simulink model "lab4"  (R2022b)
settings: Solver=VariableStepAuto  StartTime=0.0  StopTime=0.06  RelTol=1e-3
undefined symbols (not defined in the file): plecs
libraries: simulink x1, modelsimlib x1
settings Model: Creator=qawse  LastModifiedBy=qawse

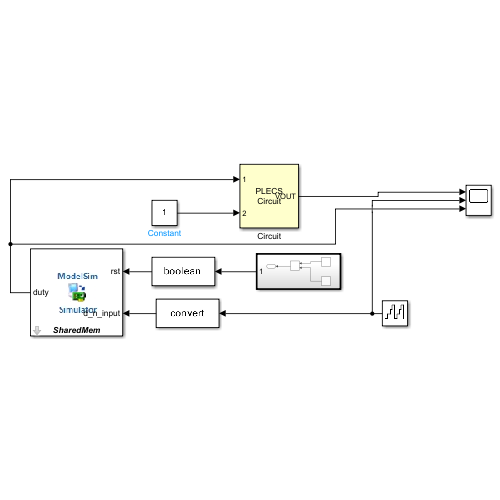
[thumbnail: Simulink's stored preview of the top-level diagram]
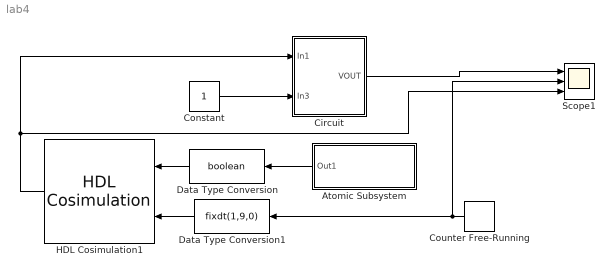
== system lab4 ==
  Atomic Subsystem : Subsystem  TreatAsAtomicUnit=on
  Circuit : Subsystem  LoadFcn=plecs('sl', 200);  InitFcn=plecs('sl', 214);  StartFcn=plecs('sl', 208);  StopFcn=plecs('sl', 209);  mask(PlecsCircuit){PLECSData=<binary blob, 2616 chars, not shown>}
      mask prompts: PLECSData "PLECS Data (Do not delete or modify!)"
      mask init:
      | % PLACE CUSTOM INITIALIZATIONS ABOVE
      | % DO NOT REMOVE
      | plecs('sl', 215);
      | % DO NOT REMOVE
      settings: CopyFcn=plecs('sl', 203);  DeleteFcn=plecs('sl', 205);  UndoDeleteFcn=plecs('sl', 206);  PreSaveFcn=plecs('sl', 211);  PostSaveFcn=plecs('sl', 201);  NameChangeFcn=plecs('sl', 210);  DestroyFcn=plecs('sl', 207);  PreCopyFcn=plecs('sl', 216);  OpenFcn=plecs('sl', 202);  ErrorFcn=plerrorfcn
      mask Help: web(['file:///' fullfile(plecsdoc, 'creatingacircuit.html')])
      mask Display: disp('PLECS\nCircuit')
  Constant : Constant
  Counter Free-Running : simulink/Sources/Counter Free-Running  NumBits=9  tsamp=1e-3
  Data Type Conversion : DataTypeConversion  OutDataTypeStr=boolean  SaturateOnIntegerOverflow=off  RndMeth=Floor
  Data Type Conversion1 : DataTypeConversion  OutDataTypeStr=fixdt(1,9,0)  SaturateOnIntegerOverflow=off  RndMeth=Floor
  HDL Cosimulation1 : modelsimlib/HDL Cosimulation  PortPaths=/counter_dpwm/rst;/counter_dpwm/d_n_input;/counter_dpwm/duty  PortModes=[1 1 2 ]  PortTimes=[-1,-1,4e-9]  PortSigns=[-1 -1 -1 ]  PortFracLengths=[0,0,0]  CommLocal=on  CommSharedMemory=on  CommPortNumber=4449  CommShowInfo=on  ClockPaths=/counter_dpwm/clk  ClockModes=[2 ]  ClockTimes=[4e-9]  TclPreSimCommand="puts \"Running Simulink Cosimulation block.\""  TclPostSimCommand="puts \"done\""  TimingMode=s  TimingScaleFactor=1  idxCellArray={'UNUSED_VAR'}  CosimBypass=Full Simulation  AllowDirectFeedthrough=off  ProductName=EDA Simulator Link MQ  RunAutoTimescale=off  HdlClocks=0  PreRunTime=0  PreRunTimeUnit=ns
  Scope1 : Scope  NumInputPorts=3
  wires:
  Circuit/1(VOUT) -> Scope1/1
  Atomic Subsystem/1(Out1) -> Data Type Conversion/1
  Counter Free-Running/1 -> Data Type Conversion1/1, Scope1/2
  Constant/1 -> Circuit/2(In3)
  Data Type Conversion/1 -> HDL Cosimulation1/1
  Data Type Conversion1/1 -> HDL Cosimulation1/2
  HDL Cosimulation1/1 -> Circuit/1(In1), Scope1/3

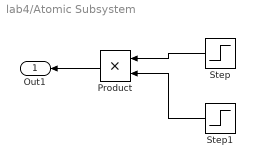
== system lab4/Atomic Subsystem ==
  Product : Product
  Step : Step  Time=1e-6  SampleTime=2e-8
  Step1 : Step  Time=1.6e-6  Before=1  After=0  SampleTime=2e-8
  Out1 : Outport
  wires:
  Product/1 -> Out1/1
  Step/1 -> Product/1
  Step1/1 -> Product/2

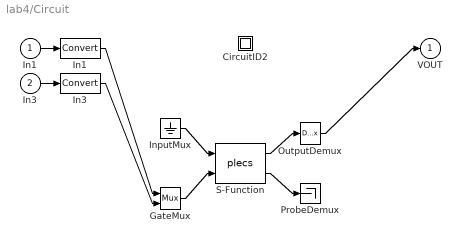
== system lab4/Circuit ==
  In1 : Inport  PortDimensions=1
  In3 : Inport  Port=2  PortDimensions=1
  " CircuitID2 " : Subsystem
  " GateMux " : Mux  Inputs=[ 1 1 ]
  " In1 " : DataTypeConversion
  " In3 " : DataTypeConversion
  " InputMux " : Ground
  " OutputDemux " : Demux  Outputs=[ 1 ]
  " ProbeDemux " : Terminator
  " S-Function " : S-Function  FunctionName=plecs  SFunctionDeploymentMode=off  EnableBusSupport=off
  VOUT : Outport  PortDimensions=1
  wires:
  " InputMux "/1 -> " S-Function "/1
  " GateMux "/1 -> " S-Function "/2
  " S-Function "/1 -> " OutputDemux "/1
  " S-Function "/2 -> " ProbeDemux "/1
  In1/1 -> " In1 "/1
  " In1 "/1 -> " GateMux "/1
  In3/1 -> " In3 "/1
  " In3 "/1 -> " GateMux "/2
  " OutputDemux "/1 -> VOUT/1

== system lab4/Circuit/ CircuitID2  ==
